simulink model "motor_anti_windup_whole_model3"  (R2019b)
settings: Solver=FixedStepAuto  StartTime=0.0  StopTime=15  FixedStep=0.001  MaxStep=0.001  RelTol=1e-5
values from neighbouring files (symbols this model uses):
  a1 = 6    [parameter_SMC_uncertainties_disturbance.m]
  b = 0.00125    [parameter_SMC_uncertainties_disturbance.m]
  Ct = 1e-8    (= 1e-08)    [parameter_SMC_uncertainties_disturbance.m]
  d1 = 0.1    [parameter_SMC_uncertainties_disturbance.m]
  d2 = 1.5    [parameter_SMC_uncertainties_disturbance.m]
  epsilon = 1    [parameter_SMC_uncertainties_disturbance.m]
  g = 9.8    [parameter_SMC_uncertainties_disturbance.m]
  J = 0.0007    [parameter_SMC_uncertainties_disturbance.m]
  Jx = 0.05    [parameter_SMC_uncertainties_disturbance.m]
  Jy = 0.08    [parameter_SMC_uncertainties_disturbance.m]
  Jz = 0.08    [parameter_SMC_uncertainties_disturbance.m]
  k_1 = 10    [parameter_SMC_uncertainties_disturbance.m]
  K_1 = 0.01    [parameter_SMC_uncertainties_disturbance.m]
  k_2 = 2.4    [parameter_SMC_uncertainties_disturbance.m]
  K_2 = 0.01    [parameter_SMC_uncertainties_disturbance.m]
  K_3 = 0.01    [parameter_SMC_uncertainties_disturbance.m]
  k_3 = 0.3    [parameter_SMC_uncertainties_disturbance.m]
  k_4 = 0.15    [parameter_SMC_uncertainties_disturbance.m]
  k_5 = 1    [parameter_SMC_uncertainties_disturbance.m]
  Kb = 0.0734    [parameter_SMC_uncertainties_disturbance.m]
  Km = 0.076    [parameter_SMC_uncertainties_disturbance.m]
  KQ = 2.925*10^-9    (= 2.925e-09)    [parameter_SMC_uncertainties_disturbance.m]
  KT = 1.4697*10^-7    (= 1.4697e-07)    [parameter_SMC_uncertainties_disturbance.m]
  l = 0.2    [parameter_SMC_uncertainties_disturbance.m]
  L = 0.000224    [parameter_SMC_uncertainties_disturbance.m]
  m = 1.5    [parameter_SMC_uncertainties_disturbance.m]
  R = 0.23    [parameter_SMC_uncertainties_disturbance.m]
  x0 = -3    [parameter_SMC_uncertainties_disturbance.m]
  y0 = -2    [parameter_SMC_uncertainties_disturbance.m]
  z0 = -2    [parameter_SMC_uncertainties_disturbance.m]
settings Model: SimulationMode=accelerator  Creator=buaaz  LastModifiedBy=nikkiy
settings GRTTargetCC: RTWCAPISignals=on  RTWCAPIParams=on

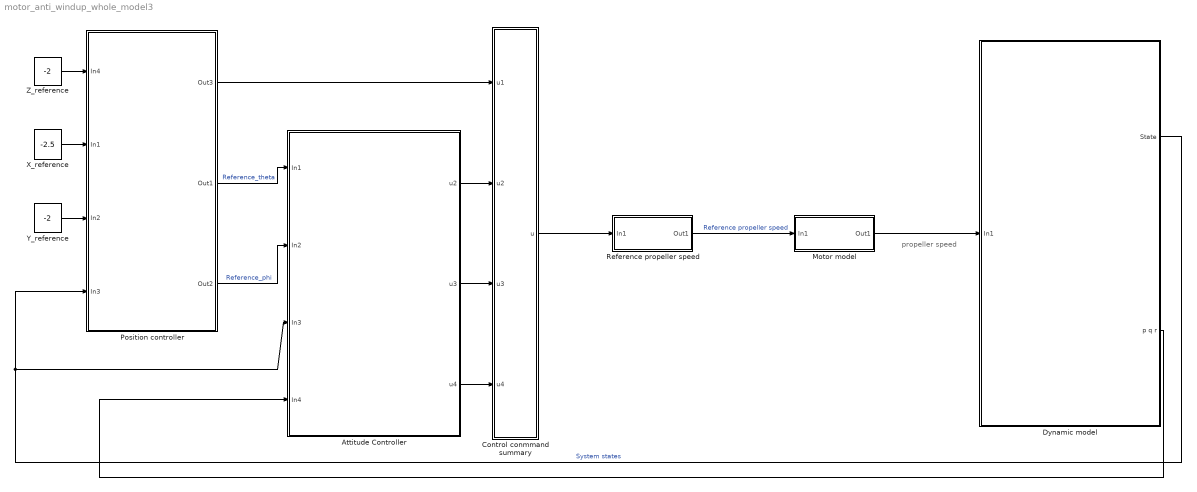
== system motor_anti_windup_whole_model3 ==
  note: propeller speed
  " X_reference" : Constant  Value=-2.5  VectorParams1D=off
  " Y_reference" : Constant  Value=-2  VectorParams1D=off
  Attitude Controller : Subsystem
  Control conmmand summary : MATLAB Function  TreatAsAtomicUnit=on
  "Dynamic model " : Subsystem
  Motor model : Subsystem
  Position controller : Subsystem
  Reference propeller speed : Subsystem
  Z_reference : Constant  Value=-2
  wires:
  Position controller/3(Out2) -> Attitude Controller/2(In2)  "Reference_phi"
  Position controller/2(Out1) -> Attitude Controller/1(In1)  "Reference_theta"
  Attitude Controller/2(u3) -> Control conmmand summary/3(u3)
  Attitude Controller/3(u4) -> Control conmmand summary/4(u4)
  Attitude Controller/1(u2) -> Control conmmand summary/2(u2)
  Position controller/1(Out3) -> Control conmmand summary/1(u1)
  " Y_reference"/1 -> Position controller/3(In2)
  " X_reference"/1 -> Position controller/2(In1)
  Z_reference/1 -> Position controller/1(In4)
  "Dynamic model "/1(State) -> Position controller/4(In3), Attitude Controller/3(In3)  "System states"
  "Dynamic model "/2(p q r) -> Attitude Controller/4(In4)
  Reference propeller speed/1(Out1) -> Motor model/1(In1)  "Reference propeller speed"
  Motor model/1(Out1) -> "Dynamic model "/1(In1)
  Control conmmand summary/1(u) -> Reference propeller speed/1(In1)

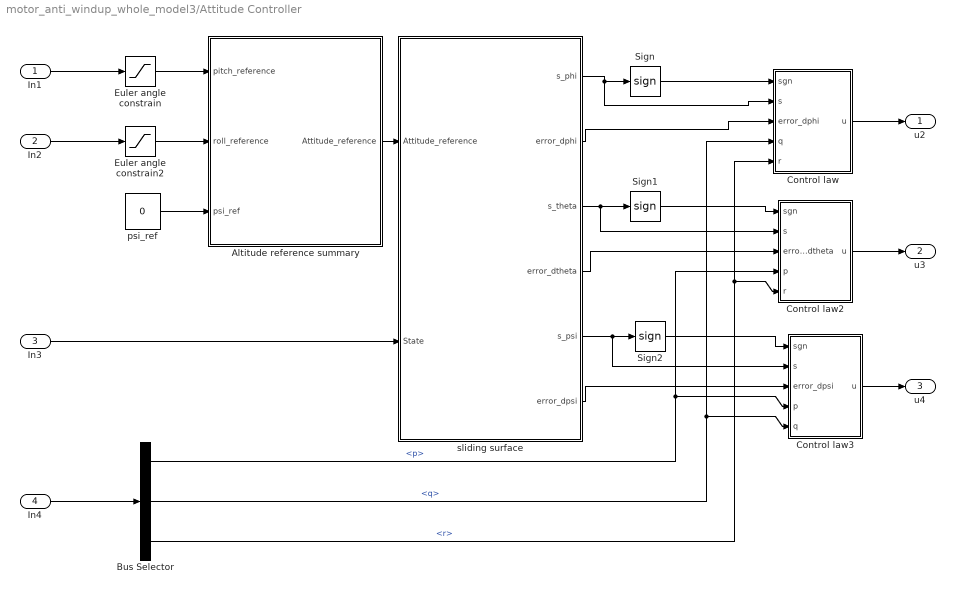
== system motor_anti_windup_whole_model3/Attitude Controller ==
  In1 : Inport
  In2 : Inport  Port=2
  In3 : Inport  Port=3
  In4 : Inport  Port=4
  Altitude reference summary : MATLAB Function  TreatAsAtomicUnit=on
  Bus Selector : BusSelector  OutputSignals=p,q,r
  Control law : MATLAB Function  TreatAsAtomicUnit=on
  Control law2 : MATLAB Function  TreatAsAtomicUnit=on
  Control law3 : MATLAB Function  TreatAsAtomicUnit=on
  Euler angle constrain : Saturate  UpperLimit=0.8  LowerLimit=-0.8
  Euler angle constrain2 : Saturate  UpperLimit=0.8  LowerLimit=-0.8
  Sign : Signum  ZeroCross=off
  Sign1 : Signum  ZeroCross=off
  Sign2 : Signum  ZeroCross=off
  psi_ref : Constant  Value=0
  sliding surface : MATLAB Function  TreatAsAtomicUnit=on
  u2 : Outport
  u3 : Outport  Port=2
  u4 : Outport  Port=3
  wires:
  sliding surface/2(error_dphi) -> Control law/3(error_dphi)
  sliding surface/4(error_dtheta) -> Control law2/3(error_dtheta)
  sliding surface/6(error_dpsi) -> Control law3/3(error_dpsi)
  sliding surface/1(s_phi) -> Sign/1, Control law/2(s)
  Sign2/1 -> Control law3/1(sgn)
  Euler angle constrain/1 -> Altitude reference summary/1(pitch_reference)
  Euler angle constrain2/1 -> Altitude reference summary/2(roll_reference)
  Sign1/1 -> Control law2/1(sgn)
  Sign/1 -> Control law/1(sgn)
  Altitude reference summary/1(Attitude_reference) -> sliding surface/1(Attitude_reference)
  sliding surface/3(s_theta) -> Sign1/1, Control law2/2(s)
  sliding surface/5(s_psi) -> Control law3/2(s), Sign2/1
  psi_ref/1 -> Altitude reference summary/3(psi_ref)
  Control law3/1(u) -> u4/1
  Control law2/1(u) -> u3/1
  Control law/1(u) -> u2/1
  In1/1 -> Euler angle constrain/1
  In2/1 -> Euler angle constrain2/1
  In3/1 -> sliding surface/2(State)
  In4/1 -> Bus Selector/1
  Bus Selector/1 -> Control law3/4(p), Control law2/4(p)  "<p>"
  Bus Selector/3 -> Control law/5(r), Control law2/5(r)  "<r>"
  Bus Selector/2 -> Control law3/5(q), Control law/4(q)  "<q>"

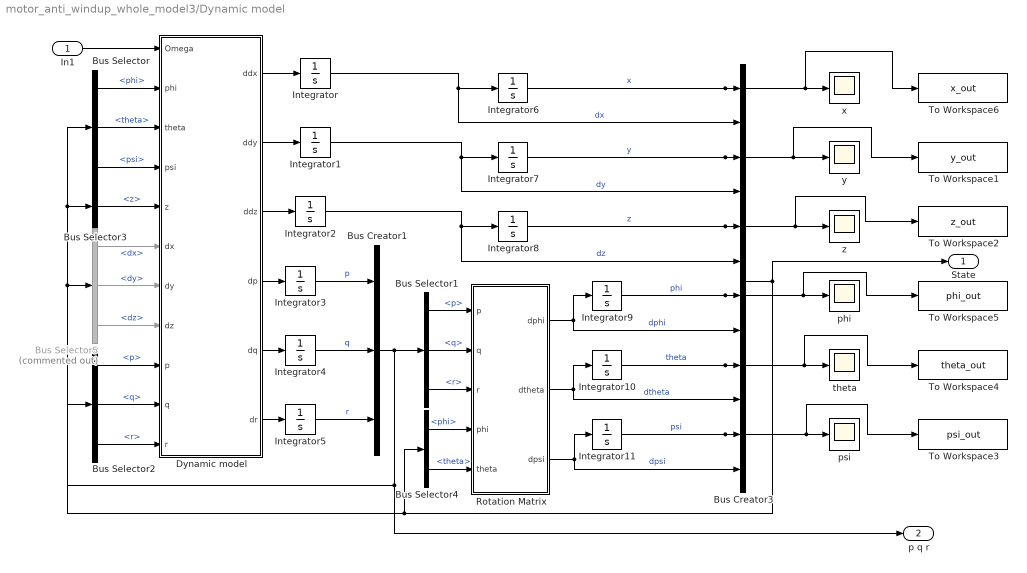
== system motor_anti_windup_whole_model3/Dynamic model  ==
  In1 : Inport
  Bus Creator1 : BusCreator  Inputs=3
  Bus Creator3 : BusCreator  Inputs=12
  Bus Selector : BusSelector  OutputSignals=phi,theta,psi
  Bus Selector1 : BusSelector  OutputSignals=p,q,r
  Bus Selector2 : BusSelector  OutputSignals=p,q,r
  Bus Selector3 : BusSelector  OutputSignals=z
  Bus Selector4 : BusSelector  OutputSignals=phi,theta
  Bus Selector5 : BusSelector  Commented=on  OutputSignals=dx,dy,dz
  Dynamic model : MATLAB Function  TreatAsAtomicUnit=on
  Integrator{,1..5,9..11} (9 alike) : Integrator
  Integrator6 : Integrator  InitialCondition=x0
  Integrator7 : Integrator  InitialCondition=y0
  Integrator8 : Integrator  InitialCondition=z0
  Rotation Matrix : MATLAB Function  TreatAsAtomicUnit=on
  To Workspace1 : ToWorkspace  VariableName=y_out  SaveFormat=Timeseries  SampleTime=-1
  To Workspace2 : ToWorkspace  VariableName=z_out  SaveFormat=Timeseries  SampleTime=-1
  To Workspace3 : ToWorkspace  VariableName=psi_out  SaveFormat=Timeseries  SampleTime=-1
  To Workspace4 : ToWorkspace  VariableName=theta_out  SaveFormat=Timeseries  SampleTime=-1
  To Workspace5 : ToWorkspace  VariableName=phi_out  SaveFormat=Timeseries  SampleTime=-1
  To Workspace6 : ToWorkspace  VariableName=x_out  SaveFormat=Timeseries  SampleTime=-1
  phi : Scope
  psi : Scope
  theta : Scope
  x : Scope
  y : Scope
  z : Scope
  State : Outport
  p q r : Outport  Port=2
  wires:
  Dynamic model/4(dp) -> Integrator3/1
  Integrator8/1 -> To Workspace2/1, z/1, Bus Creator3/5  "z"
  Bus Selector4/1 -> Rotation Matrix/4(phi)  "<phi>"
  Bus Selector5/1 -> Dynamic model/6(dx)  "<dx>"
  Integrator2/1 -> Bus Creator3/6, Integrator8/1  "dz"
  Bus Selector5/2 -> Dynamic model/7(dy)  "<dy>"
  Dynamic model/1(ddx) -> Integrator/1
  Bus Selector1/2 -> Rotation Matrix/2(q)  "<q>"
  Integrator9/1 -> Bus Creator3/7, To Workspace5/1, phi/1  "phi"
  Bus Selector1/3 -> Rotation Matrix/3(r)  "<r>"
  Dynamic model/5(dq) -> Integrator4/1
  Integrator7/1 -> To Workspace1/1, y/1, Bus Creator3/3  "y"
  Integrator4/1 -> Bus Creator1/2  "q"
  Integrator3/1 -> Bus Creator1/1  "p"
  Rotation Matrix/3(dpsi) -> Bus Creator3/12, Integrator11/1  "dpsi"
  Integrator/1 -> Bus Creator3/2, Integrator6/1  "dx"
  Bus Selector/1 -> Dynamic model/2(phi)  "<phi>"
  Dynamic model/6(dr) -> Integrator5/1
  Bus Selector2/1 -> Dynamic model/9(p)  "<p>"
  Integrator5/1 -> Bus Creator1/3  "r"
  Dynamic model/2(ddy) -> Integrator1/1
  Integrator1/1 -> Bus Creator3/4, Integrator7/1  "dy"
  Bus Selector2/3 -> Dynamic model/11(r)  "<r>"
  In1/1 -> Dynamic model/1(Omega)
  Bus Selector4/2 -> Rotation Matrix/5(theta)  "<theta>"
  Bus Selector5/3 -> Dynamic model/8(dz)  "<dz>"
  Bus Creator1/1 -> Bus Selector1/1, Bus Selector2/1, p q r/1
  Bus Selector/2 -> Dynamic model/3(theta)  "<theta>"
  Bus Selector/3 -> Dynamic model/4(psi)  "<psi>"
  Bus Selector1/1 -> Rotation Matrix/1(p)  "<p>"
  Dynamic model/3(ddz) -> Integrator2/1
  Bus Selector2/2 -> Dynamic model/10(q)  "<q>"
  Rotation Matrix/1(dphi) -> Bus Creator3/8, Integrator9/1  "dphi"
  Integrator6/1 -> To Workspace6/1, x/1, Bus Creator3/1  "x"
  Bus Creator3/1 -> State/1, Bus Selector4/1, Bus Selector5/1, Bus Selector3/1, Bus Selector/1
  Integrator10/1 -> Bus Creator3/9, To Workspace4/1, theta/1  "theta"
  Integrator11/1 -> Bus Creator3/11, To Workspace3/1, psi/1  "psi"
  Rotation Matrix/2(dtheta) -> Bus Creator3/10, Integrator10/1  "dtheta"
  Bus Selector3/1 -> Dynamic model/5(z)  "<z>"

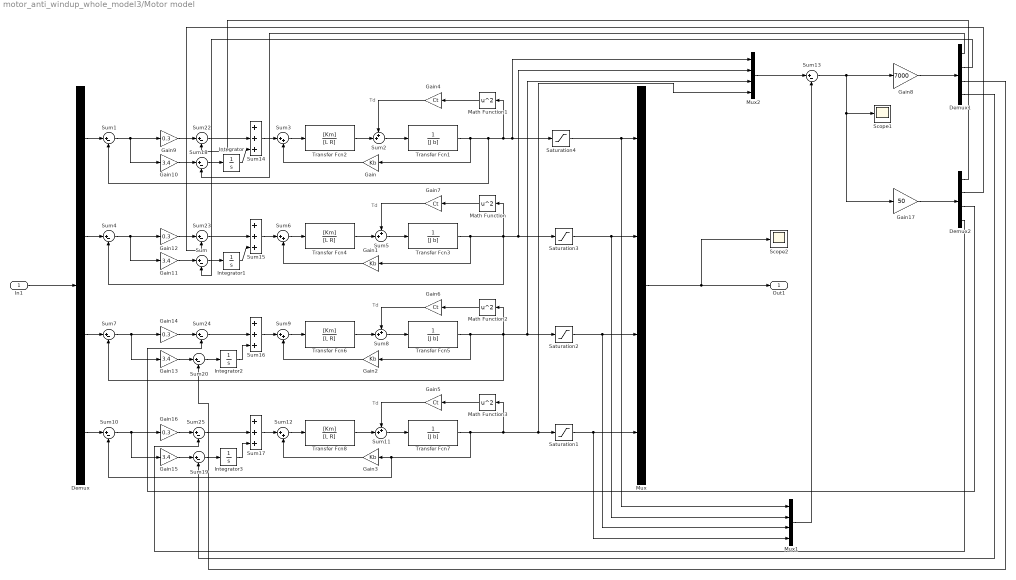
== system motor_anti_windup_whole_model3/Motor model ==
  note: Td
  note: Td
  note: Td
  note: Td
  In1 : Inport
  Demux : Demux
  Demux1 : Demux
  Demux2 : Demux
  Gain{,1..3} (4 alike) : Gain  Gain=Kb
  Gain{10..11,13,15} (4 alike) : Gain  Gain=3.4
  Gain{9,12,14,16} (4 alike) : Gain  Gain=0.3
  Gain17 : Gain  Gain=50
  Gain{4..7} (4 alike) : Gain  Gain=Ct
  Gain8 : Gain  Gain=7000
  Integrator{,1..3} (4 alike) : Integrator
  Math Function{,1..3} (4 alike) : Math  Operator=square  SignedPower=off  SaturateOnIntegerOverflow=on
  Mux : Mux
  Mux1 : Mux
  Mux2 : Mux
  Saturation{1..4} (4 alike) : Saturate  UpperLimit=6200  LowerLimit=0
  Scope1 : Scope
  Scope2 : Scope
  Sum{,1,4,7,10,13,18..20,22..25} (13 alike) : Sum  Inputs=|+-
  Sum{2,5,8,11} (4 alike) : Sum  Inputs=++|
  Sum{3,6,9,12} (4 alike) : Sum  Inputs=|++
  Sum{14..17} (4 alike) : Sum  Inputs=+++
  Transfer Fcn{1,3,5,7} (4 alike) : TransferFcn  Denominator=[J b]
  Transfer Fcn{2,4,6,8} (4 alike) : TransferFcn  Numerator=[Km]  Denominator=[L R]
  Out1 : Outport
  wires:
  Sum1/1 -> Gain9/1, Gain10/1
  Transfer Fcn2/1 -> Sum2/2
  Gain4/1 -> Sum2/1
  Sum2/1 -> Transfer Fcn1/1
  Sum14/1 -> Sum3/1
  Sum3/1 -> Transfer Fcn2/1
  Gain/1 -> Sum3/2
  Mux/1 -> Scope2/1, Out1/1
  Sum6/1 -> Transfer Fcn4/1
  Gain7/1 -> Sum5/1
  Gain1/1 -> Sum6/2
  Transfer Fcn4/1 -> Sum5/2
  Sum5/1 -> Transfer Fcn3/1
  Sum9/1 -> Transfer Fcn6/1
  Sum16/1 -> Sum9/1
  Gain6/1 -> Sum8/1
  Gain2/1 -> Sum9/2
  Transfer Fcn6/1 -> Sum8/2
  Sum8/1 -> Transfer Fcn5/1
  Sum12/1 -> Transfer Fcn8/1
  Gain5/1 -> Sum11/1
  Gain3/1 -> Sum12/2
  Transfer Fcn8/1 -> Sum11/2
  Demux/4 -> Sum10/1
  Sum11/1 -> Transfer Fcn7/1
  Math Function1/1 -> Gain4/1
  Math Function2/1 -> Gain6/1
  Math Function/1 -> Gain7/1
  Math Function3/1 -> Gain5/1
  Saturation2/1 -> Mux1/3, Mux/3
  Saturation3/1 -> Mux1/2, Mux/2
  Saturation4/1 -> Mux1/1, Mux/1
  Mux1/1 -> Sum13/2
  Saturation1/1 -> Mux1/4, Mux/4
  Transfer Fcn1/1 -> Mux2/1, Saturation4/1, Math Function1/1, Sum1/2, Gain/1
  Transfer Fcn3/1 -> Sum4/2, Mux2/2, Saturation3/1, Math Function/1, Gain1/1
  Transfer Fcn5/1 -> Mux2/3, Saturation2/1, Sum7/2, Math Function2/1, Gain2/1
  Transfer Fcn7/1 -> Sum10/2, Gain3/1, Mux2/4, Saturation1/1, Math Function3/1
  Mux2/1 -> Sum13/1
  Sum13/1 -> Gain17/1, Scope1/1, Gain8/1
  Sum4/1 -> Gain12/1, Gain11/1
  Sum15/1 -> Sum6/1
  Integrator2/1 -> Sum16/3
  Sum7/1 -> Gain14/1, Gain13/1
  Sum10/1 -> Gain16/1, Gain15/1
  Integrator3/1 -> Sum17/3
  Sum17/1 -> Sum12/1
  Demux/1 -> Sum1/1
  Demux/2 -> Sum4/1
  Demux/3 -> Sum7/1
  Gain13/1 -> Sum20/1
  Sum20/1 -> Integrator2/1
  Gain11/1 -> Sum/1
  Sum/1 -> Integrator1/1
  Gain10/1 -> Sum18/1
  Sum18/1 -> Integrator/1
  Gain15/1 -> Sum19/1
  Sum19/1 -> Integrator3/1
  Demux1/1 -> Sum18/2
  Demux1/2 -> Sum/2
  Demux1/3 -> Sum20/2
  Demux1/4 -> Sum19/2
  Integrator/1 -> Sum14/3
  Integrator1/1 -> Sum15/3
  In1/1 -> Demux/1
  Gain8/1 -> Demux1/1
  Gain9/1 -> Sum22/1
  Sum22/1 -> Sum14/2
  Gain12/1 -> Sum23/1
  Sum23/1 -> Sum15/2
  Gain14/1 -> Sum24/1
  Sum24/1 -> Sum16/2
  Gain16/1 -> Sum25/1
  Sum25/1 -> Sum17/2
  Demux2/1 -> Sum22/2
  Demux2/2 -> Sum23/2
  Demux2/3 -> Sum24/2
  Demux2/4 -> Sum25/2
  Gain17/1 -> Demux2/1

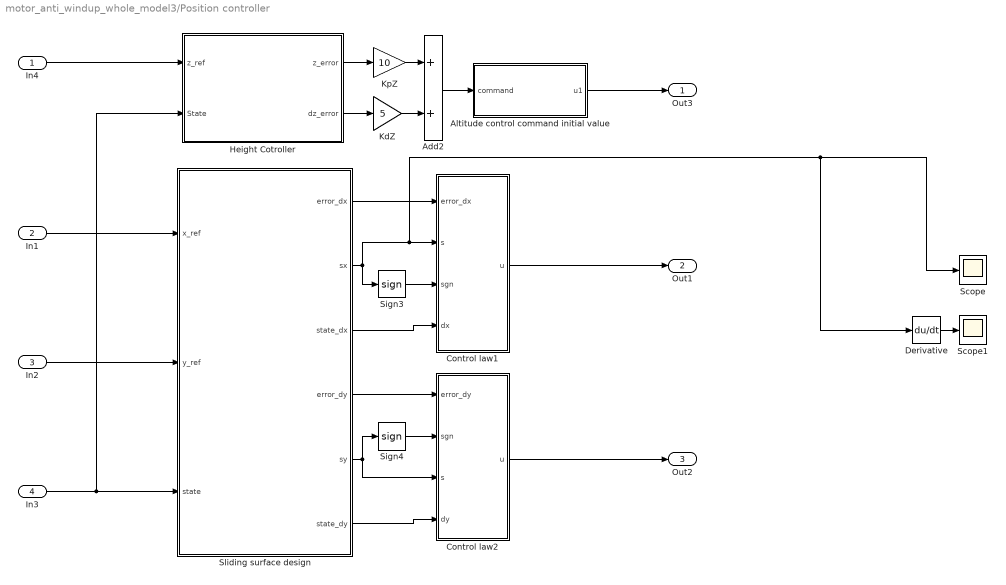
== system motor_anti_windup_whole_model3/Position controller ==
  In4 : Inport
  In1 : Inport  Port=2
  In2 : Inport  Port=3
  In3 : Inport  Port=4
  Add2 : Sum
  Altitude control command initial value : MATLAB Function  TreatAsAtomicUnit=on
  Control law1 : MATLAB Function  TreatAsAtomicUnit=on
  Control law2 : MATLAB Function  TreatAsAtomicUnit=on
  Derivative : Derivative
  Height Cotroller : MATLAB Function  TreatAsAtomicUnit=on
  KdZ : Gain  Gain=5
  KpZ : Gain  Gain=10
  Scope : Scope
  Scope1 : Scope
  Sign3 : Signum  ZeroCross=off
  Sign4 : Signum  ZeroCross=off
  Sliding surface design : MATLAB Function  TreatAsAtomicUnit=on
  Out3 : Outport
  Out1 : Outport  Port=2
  Out2 : Outport  Port=3
  wires:
  Sliding surface design/6(state_dy) -> Control law2/4(dy)
  Sliding surface design/5(sy) -> Control law2/3(s), Sign4/1
  Sliding surface design/4(error_dy) -> Control law2/1(error_dy)
  Sliding surface design/3(state_dx) -> Control law1/4(dx)
  Sign4/1 -> Control law2/2(sgn)
  Sliding surface design/1(error_dx) -> Control law1/1(error_dx)
  Sign3/1 -> Control law1/3(sgn)
  Add2/1 -> Altitude control command initial value/1(command)
  Height Cotroller/2(dz_error) -> KdZ/1
  KpZ/1 -> Add2/1
  Height Cotroller/1(z_error) -> KpZ/1
  KdZ/1 -> Add2/2
  Control law1/1(u) -> Out1/1
  Control law2/1(u) -> Out2/1
  In1/1 -> Sliding surface design/1(x_ref)
  In3/1 -> Height Cotroller/2(State), Sliding surface design/3(state)
  In2/1 -> Sliding surface design/2(y_ref)
  In4/1 -> Height Cotroller/1(z_ref)
  Altitude control command initial value/1(u1) -> Out3/1
  Sliding surface design/2(sx) -> Derivative/1, Scope/1, Control law1/2(s), Sign3/1
  Derivative/1 -> Scope1/1

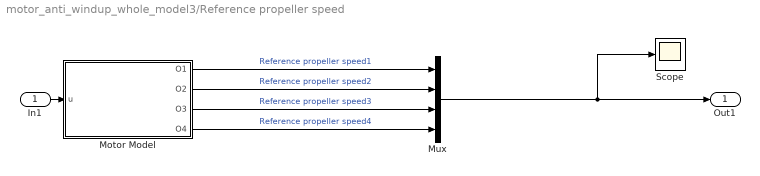
== system motor_anti_windup_whole_model3/Reference propeller speed ==
  In1 : Inport
  Motor Model : MATLAB Function  TreatAsAtomicUnit=on
  Mux : Mux
  Scope : Scope
  Out1 : Outport
  wires:
  Motor Model/2(O2) -> Mux/2  "Reference propeller speed2"
  Motor Model/3(O3) -> Mux/3  "Reference propeller speed3"
  Motor Model/4(O4) -> Mux/4  "Reference propeller speed4"
  In1/1 -> Motor Model/1(u)
  Motor Model/1(O1) -> Mux/1  "Reference propeller speed1"
  Mux/1 -> Scope/1, Out1/1

== matlab function motor_anti_windup_whole_model3/Control conmmand summary ==
  data: u output; u1 input double; u2 input double; u3 input double; u4 input
function u = fcn(u1,u2, u3,u4)
u=[u1 u2 u3 u4]

== matlab function motor_anti_windup_whole_model3/Attitude Controller/sliding surface ==
  data: Attitude_reference input double; State input; s_phi output double; error_dphi output; s_theta output double; error_dtheta output; s_psi output double; error_dpsi output; a1 parameter; epsilon parameter
function [s_phi,error_dphi,s_theta,error_dtheta,s_psi,error_dpsi]  = fcn(Attitude_reference,State,a1, epsilon)
dAttitude_redernce=[0 0 0]
State1=[State(7) State(9) State(11)]                   %Euler angle
State2=[State(8) State(10) State(12)]                 %dEuler angle

Error_vector1=State1-Attitude_reference           %Euler angle error
Error_vector2=State2-dAttitude_redernce           %dEuler angle error

error_phi=Error_vector1(1)
error_dphi=Error_vector2(1)
error_theta=Error_vector1(2)
error_dtheta=Error_vector2(2)
error_psi=Error_vector1(3)
error_dpsi=Error_vector2(3)

%sliding surface design
s_phi=(a1*error_phi+error_dphi)/epsilon
s_theta=(a1*error_theta+error_dtheta)/epsilon
s_psi=(a1*error_psi+error_dpsi)/epsilon

== matlab function motor_anti_windup_whole_model3/Attitude Controller/Control law2 ==
  data: sgn input; s input; k_2 parameter; error_dtheta input; k_1 parameter; u output; p input; r input; k_5 parameter; Jx parameter; Jz parameter
function u = fcn( sgn,s,k_2,error_dtheta, k_1,p,r,k_5, Jx, Jz)
if  abs(s)< 0.5
u= -k_1*s-k_2*error_dtheta-k_5*abs(p)*abs(r)*(Jx-Jz)*sgn
else
u= -k_1*sgn-k_2*error_dtheta-k_5*abs(p)*abs(r)*(Jx-Jz)*sgn
end

== matlab function motor_anti_windup_whole_model3/Attitude Controller/Control law ==
  data: u output; sgn input; s input; k_2 parameter; error_dphi input; k_1 parameter; epsilon parameter; q input; r input; k_5 parameter; Jy parameter; Jz parameter
function u = fcn( sgn,s,k_2,error_dphi, k_1, epsilon,q,r,k_5, Jy, Jz)
if  abs(s)< epsilon
u= -k_1*s-k_2*error_dphi-k_5*abs(q)*abs(r)*(Jz-Jy)*sgn
else
u= -k_1*sgn-k_2*error_dphi-k_5*abs(q)*abs(r)*(Jz-Jy)*sgn
end

== matlab function motor_anti_windup_whole_model3/Attitude Controller/Control law3 ==
  data: u output; sgn input; s input; k_2 parameter; error_dpsi input; k_1 parameter; p input; q input; k_5 parameter; Jx parameter; Jy parameter
function u = fcn( sgn,s,k_2,error_dpsi, k_1,p,q,k_5, Jx, Jy)
if  abs(s)< 0.5
u= -k_1*s-k_2*error_dpsi-k_5*abs(p)*abs(q)*(Jy-Jx)*sgn
else
u= -k_1*sgn-k_2*error_dpsi-k_5*abs(p)*abs(q)*(Jy-Jx)*sgn
end

== matlab function motor_anti_windup_whole_model3/Position controller/Control law1 ==
  data: error_dx input; s input; u output; K_1 parameter; k_3 parameter; k_4 parameter; sgn input; dx input
 function u   = fcn(error_dx,s,K_1, k_3,k_4,sgn, dx)
u=k_3*s-k_4*abs(error_dx)+K_1*dx/9.8
end

== matlab function motor_anti_windup_whole_model3/Position controller/Control law2 ==
  data: error_dy input; u output; sgn input double; k_4 parameter; k_3 parameter; K_1 parameter; s input; dy input
 function u   = fcn(error_dy,sgn, k_4, k_3, K_1, s,dy)
u=-k_3*s+k_4*abs(error_dy)-K_1*dy/9.8
end

== matlab function motor_anti_windup_whole_model3/Position controller/Height Cotroller ==
  data: z_ref input; State input; z_error output; dz_error output
function [z_error,dz_error] = fcn(z_ref,State)
dz_ref=0
z_error=State(5)-z_ref
dz_error=State(6)-dz_ref

== matlab function motor_anti_windup_whole_model3/Attitude Controller/Altitude reference summary ==
  data: pitch_reference input double; roll_reference input double; psi_ref input; Attitude_reference output double
function Attitude_reference  = fcn(pitch_reference,roll_reference, psi_ref)
Attitude_reference=[roll_reference pitch_reference psi_ref]
% Attitude_reference=[0 0.4 0]

== matlab function motor_anti_windup_whole_model3/Position controller/Altitude control command initial value ==
  data: u1 output; command input; m parameter; g parameter
function u1 = fcn(command, m, g)
u1=m*g+command

%This is an initial command of the altitude controller, because we assume
% the drone is hovering.

%If we want begin on the ground, please use the following control laws
%u1=command

== matlab function motor_anti_windup_whole_model3/Position controller/Sliding surface design ==
  data: error_dx output; x_ref input; y_ref input; state input size=12; sx output; state_dx output; error_dy output; sy output; state_dy output; a2 parameter
function [error_dx,sx,state_dx,error_dy,sy,state_dy] = fcn(x_ref,y_ref,state,a2)
state_x=state(1)
state_dx=state(2)
state_y=state(3)
state_dy=state(4)

error_x=state_x-x_ref
error_y=state_y-y_ref

error_dy=state_dy-0
error_dx=state_dx-0
%sliding surface design
sx=a2*error_x+error_dx
sy=a2*error_y+error_dy
end

== matlab function motor_anti_windup_whole_model3/Dynamic model /Dynamic model ==
  data: Omega input double; ddx output size=1; phi input; theta input; psi input; KQ parameter; KT parameter; l parameter; g parameter; z input; dx input; dy input; dz input; p input; q input; r input; Jy parameter; Jz parameter; Jx parameter; m parameter; ddy output size=1; ddz output size=1; dp output size=1; dq output size=1; dr output size=1; K_1 parameter; K_2 parameter; K_3 parameter; d1 parameter; d2 parameter
 function [ddx,ddy,ddz,dp,dq,dr] = fcn(Omega,phi,theta,psi,KQ, KT,l,g,z,dx,dy,dz,p,q,r, Jy, Jz, Jx, m,K_1,K_2,K_3,d1,d2)
 
%propeller speed
 O1=Omega(1);
O2=Omega(2);
O3=Omega(3);
O4=Omega(4);

%The dynamic model is divided into three cases based on ground effect

%Altitude without ground effect
if z<-2*l
ddx=(sin(phi).*sin(psi)+cos(phi).*sin(theta).*cos(psi)).*(-KT.*(O1^2+O2^2+O3^2+O4^2))/m-(K_1*dx)/m+d1
ddy=(-sin(phi).*cos(psi)+cos(phi).*sin(theta).*sin(psi)).*(-KT.*(O1^2+O2^2+O3^2+O4^2))/m-(K_2*dy)/m
ddz=g+(cos(phi).*cos(theta)).*(-KT.*(O1^2+O2^2+O3^2+O4^2))/m-(K_3*dz)/m
dp=(l.*KT.*(O1^2+O4^2-O2^2-O3^2)-q.*r*(Jz-Jy))/Jx
dq=(l.*KT.*(O2^2+O4^2-O1^2-O3^2)-p.*r*(Jx-Jz))/Jy+d2
dr=(l.*KQ.*(-O1^2-O2^2+O3^2+O4^2)-p.*q.*(Jy-Jx))/Jz

%Altitude affected by ground effects
else if  z<0&z>-2*l&z==-2*l
ddx=(sin(phi).*sin(psi)+cos(phi).*sin(theta).*cos(psi)).*(-KT.*(O1^2+O2^2+O3^2+O4^2))/m-(K_1*dx)/m+d1
ddy=(-sin(phi).*cos(psi)+cos(phi).*sin(theta).*sin(psi)).*(-KT.*(O1^2+O2^2+O3^2+O4^2))/m-(K_2*dy)/m
ddz=g+(2.6-1.6*(-z/2*l))*(cos(phi).*cos(theta)).*(-KT.*(O1^2+O2^2+O3^2+O4^2))/m-(K_3*dz)/m
dp=(l.*KT.*(O1^2+O4^2-O2^2-O3^2)-q.*r*(Jz-Jy))/Jx
dq=(l.*KT.*(O2^2+O4^2-O1^2-O3^2)-p.*r*(Jx-Jz))/Jy+d2
dr=(l.*KQ.*(-O1^2-O2^2+O3^2+O4^2)-p.*q.*(Jy-Jx))/Jz

%After the drone crashed
else
ddx=0
ddy=0
ddz=0
dp=0
dq=0
dr=0
    end
end

== matlab function motor_anti_windup_whole_model3/Dynamic model /Rotation Matrix ==
  data: p input; dphi output; dtheta output; dpsi output; q input; r input; phi input; theta input
function [dphi,dtheta,dpsi] = fcn(p,q,r,phi,theta)
dphi=p+q*sin(phi)*tan(theta)+r*cos(phi)*tan(theta)
dtheta=q*cos(phi)-r*sin(phi)
dpsi=q*sin(phi)/cos(theta)+r*cos(phi)/cos(theta)
% dphi=p
% dtheta=q
% dpsi=r

== matlab function motor_anti_windup_whole_model3/Reference propeller speed/Motor Model ==
  data: u input double; O1 output; O2 output; O3 output; O4 output; KQ parameter; KT parameter; l parameter
function [O1,O2,O3,O4] = fcn(u,KQ, KT,l)
u1=u(1)
u2=u(2)
u3=u(3)
u4=u(4)

%re-calculate matrix
R=[KT KT KT KT;...
   KT -KT -KT KT;...
   -KT KT -KT KT;...
   -KQ*l -KQ*l KQ*l KQ*l]

%propeller speed must greater than 0
OMEGA=inv(R)*[u1;u2;u3;u4]
if OMEGA(1)<=0
    OMEGA(1)=0
else
    OMEGA(1)=OMEGA(1)
end
if OMEGA(2)<=0
    OMEGA(2)=0
else
    OMEGA(2)=OMEGA(2)
end
if OMEGA(3)<=0
    OMEGA(3)=0
else
    OMEGA(3)=OMEGA(3)
end
if OMEGA(4)<=0
    OMEGA(4)=0
else
    OMEGA(4)=OMEGA(4)
end

%propeller speed
O1=sqrt(OMEGA(1)) 
O2=sqrt(OMEGA(2))
O3=sqrt(OMEGA(3))
O4=sqrt(OMEGA(4))
